simulink model "CCH_simulink"  (R2023a)
settings: Solver=VariableStepAuto  StartTime=0.0  StopTime=10.0  RelTol=1e-3
model workspace (MAT data in the model file):
  op_trim1 = opcond.OperatingReport
  op_trim1.Outputs_(1) = opcond.OutputReport
  op_trim1.Outputs_(1).yspec_ = 0
  op_trim1.Outputs_(1).Block_ = 'untitled1/Output'
  op_trim1.Outputs_(1).PortWidth_ = 1
  op_trim1.Outputs_(1).PortNumber_ = NaN
  op_trim1.Outputs_(1).Known_ = 0
  op_trim1.Outputs_(1).Min_ = -Inf
  op_trim1.Outputs_(1).Max_ = Inf
  op_trim1.Outputs_(2) = opcond.OutputReport
  op_trim1.Outputs_(2).yspec_ = 0
  op_trim1.Outputs_(2).Block_ = 'untitled1/Output1'
  op_trim1.Outputs_(2).PortWidth_ = 1
  op_trim1.Outputs_(2).PortNumber_ = NaN
  op_trim1.Outputs_(2).Known_ = 0
  op_trim1.Outputs_(2).Min_ = -Inf
  op_trim1.Outputs_(2).Max_ = Inf
  op_trim1.Outputs_(3) = opcond.OutputReport
  op_trim1.Outputs_(3).yspec_ = 0
  op_trim1.Outputs_(3).Block_ = 'untitled1/Output2'
  op_trim1.Outputs_(3).PortWidth_ = 1
  op_trim1.Outputs_(3).PortNumber_ = NaN
  op_trim1.Outputs_(3).Known_ = 0
  op_trim1.Outputs_(3).Min_ = -Inf
  op_trim1.Outputs_(3).Max_ = Inf
  op_trim1.Outputs_(4) = opcond.OutputReport
  op_trim1.Outputs_(4).yspec_ = 0
  op_trim1.Outputs_(4).Block_ = 'untitled1/Output3'
  op_trim1.Outputs_(4).PortWidth_ = 1
  op_trim1.Outputs_(4).PortNumber_ = NaN
  op_trim1.Outputs_(4).Known_ = 0
  op_trim1.Outputs_(4).Min_ = -Inf
  op_trim1.Outputs_(4).Max_ = Inf
  op_trim1.Outputs_(5) = opcond.OutputReport
  op_trim1.Outputs_(5).yspec_ = 0
  op_trim1.Outputs_(5).Block_ = 'untitled1/Output4'
  op_trim1.Outputs_(5).PortWidth_ = 1
  op_trim1.Outputs_(5).PortNumber_ = NaN
  op_trim1.Outputs_(5).Known_ = 0
  op_trim1.Outputs_(5).Min_ = -Inf
  op_trim1.Outputs_(5).Max_ = Inf
  op_trim1.TerminationString_ = 'Operating point specifications were successfully met.'
  op_trim1.OptimizationOutput_.iterations = 9
  op_trim1.OptimizationOutput_.funcCount = 115
  op_trim1.OptimizationOutput_.lssteplength = 1
  op_trim1.OptimizationOutput_.stepsize = 6.70795164914e-07
  op_trim1.OptimizationOutput_.algorithm = 'active-set'
  op_trim1.OptimizationOutput_.firstorderopt = 0
  op_trim1.OptimizationOutput_.constrviolation = 4.6916004894e-07
  op_trim1.OptimizationOutput_.message = 'Local minimum found that satisfies the constraints.
    | 
    | Optimization completed because the objective function is non-decreasing in 
    | feasible directions, to within the value of the optimality tolerance,
    | and constraints are satisfied to within the  value of the constraint tolerance.
    | 
    | <stopping criteria details>
    | 
    | Optimization completed: The first-order optimality measure, 0.000000e+00, is less
    | than options.OptimalityTolerance = 1.000000e-06, and the maximum constraint violation,
    | 4.691600e-07,is less than options.ConstraintTolerance = 1.000000e-06.'
  op_trim1.OptimizationOutput_.bestfeasible.x = [0.00151783990311; 0.004754547464; 0.000128910185441; 0.0400087459164; -0.0616136742271; -0.0892807825145; 0.340864918915; -3.49524304204e-06; 0.0478268463383]
  op_trim1.OptimizationOutput_.bestfeasible.fval = 0
  op_trim1.OptimizationOutput_.bestfeasible.constrviolation = 4.6916004894e-07
  op_trim1.OptimizationOutput_.bestfeasible.firstorderopt = 0
  op_trim1.OptimizationOutput_.progress = {'<font face="monospaced"; size=3><BR>', 'Optimizing to solve for all desired dx/dt=0, x(k+1)-x(k)=0, and y=ydes.<BR>', ' <BR>', '(Maximum Error)  Block<BR>', ' ---------------------------------------------------------<BR>', '(1.83311e+01) untitled1/CCH Dynamics/w<BR>', '(1.83310e+01) untitled1/CCH Dynamics/w<BR>', '(3.33587e+00) untitled1/CCH Dynamics/lambda_0_u<BR>', '(8.26009e-01) untitled1/CCH Dynamics/lambda_0_u<BR>', '(1.98820e-01) untitled1/CCH Dynamics/lambda_0_u<BR>', '(4.28137e-02) untitled1/CCH Dynamics/lambda_0_u<BR>', '(6.12506e-03) untitled1/CCH Dynamics/lambda_0_u<BR>', '(2.45994e-04) untitled1/CCH Dynamics/lambda_0_u<BR>', '(4.69160e-07) untitled1/CCH Dynamics/lambda_0_u<BR>', '(4.69160e-07) untitled1/CCH Dynamics/lambda_0_u<BR>', ' <BR>', 'Operating point specifications were successfully met.<BR>'}
  op_trim1.Model_ = 'untitled1'
  op_trim1.States_(1) = opcond.StateReport
  op_trim1.States_(1).dx_ = -2.49032220193e-09
  op_trim1.States_(1).Nx_ = 1
  op_trim1.States_(1).Block_ = 'untitled1/CCH Dynamics/lambda_0_p'
  op_trim1.States_(1).x_ = -0.0616136742271
  op_trim1.States_(1).SteadyState_ = 1
  op_trim1.States_(1).dxMin_ = -Inf
  op_trim1.States_(1).dxMax_ = Inf
  op_trim1.States_(1).Known_ = 0
  op_trim1.States_(1).Min_ = -Inf
  op_trim1.States_(1).Max_ = Inf
  op_trim1.States_(2) = opcond.StateReport
  op_trim1.States_(2).dx_ = -4.6916004894e-07
  op_trim1.States_(2).Nx_ = 1
  op_trim1.States_(2).Block_ = 'untitled1/CCH Dynamics/lambda_0_u'
  op_trim1.States_(2).x_ = 0.0400087459164
  op_trim1.States_(2).SteadyState_ = 1
  op_trim1.States_(2).dxMin_ = -Inf
  op_trim1.States_(2).dxMax_ = Inf
  op_trim1.States_(2).Known_ = 0
  op_trim1.States_(2).Min_ = -Inf
  op_trim1.States_(2).Max_ = Inf
  op_trim1.States_(3) = opcond.StateReport
  op_trim1.States_(3).dx_ = -3.96070598844e-12
  op_trim1.States_(3).Nx_ = 1
  op_trim1.States_(3).Block_ = 'untitled1/CCH Dynamics/q'
  op_trim1.States_(3).x_ = 0.000128910185441
  op_trim1.States_(3).SteadyState_ = 1
  op_trim1.States_(3).dxMin_ = -Inf
  op_trim1.States_(3).dxMax_ = Inf
  op_trim1.States_(3).Known_ = 0
  op_trim1.States_(3).Min_ = -Inf
  op_trim1.States_(3).Max_ = Inf
  op_trim1.States_(4) = opcond.StateReport
  op_trim1.States_(4).dx_ = 0.000128910185441
  op_trim1.States_(4).Nx_ = 1
  op_trim1.States_(4).Block_ = 'untitled1/CCH Dynamics/theta_f'
  op_trim1.States_(4).x_ = -0.0892807825145
  op_trim1.States_(4).SteadyState_ = 0
  op_trim1.States_(4).dxMin_ = -Inf
  op_trim1.States_(4).dxMax_ = Inf
  op_trim1.States_(4).Known_ = 0
  op_trim1.States_(4).Min_ = -Inf
  op_trim1.States_(4).Max_ = Inf
  op_trim1.States_(5) = opcond.StateReport
  op_trim1.States_(5).dx_ = -3.38404100297e-08
  op_trim1.States_(5).Nx_ = 1
  op_trim1.States_(5).Block_ = 'untitled1/CCH Dynamics/u'
  op_trim1.States_(5).x_ = 0.00151783990311
  op_trim1.States_(5).SteadyState_ = 1
  op_trim1.States_(5).dxMin_ = -Inf
  op_trim1.States_(5).dxMax_ = Inf
  op_trim1.States_(5).Known_ = 0
  op_trim1.States_(5).Min_ = -Inf
  op_trim1.States_(5).Max_ = Inf
  op_trim1.States_(6) = opcond.StateReport
  op_trim1.States_(6).dx_ = -9.51930090309e-10
  op_trim1.States_(6).Nx_ = 1
  op_trim1.States_(6).Block_ = 'untitled1/CCH Dynamics/w'
  op_trim1.States_(6).x_ = 0.004754547464
  op_trim1.States_(6).SteadyState_ = 1
  op_trim1.States_(6).dxMin_ = -Inf
  op_trim1.States_(6).dxMax_ = Inf
  op_trim1.States_(6).Known_ = 0
  op_trim1.States_(6).Min_ = -Inf
  op_trim1.States_(6).Max_ = Inf
  op_trim1.Inputs_(1) = opcond.InputReport
  op_trim1.Inputs_(1).Block_ = 'untitled1/Coll'
  op_trim1.Inputs_(1).PortWidth_ = 1
  op_trim1.Inputs_(1).PortDimensions_ = [1 1]
  op_trim1.Inputs_(1).u_ = 0.340864918915
  op_trim1.Inputs_(1).Known_ = 0
  op_trim1.Inputs_(1).Min_ = -Inf
  op_trim1.Inputs_(1).Max_ = Inf
  op_trim1.Inputs_(2) = opcond.InputReport
  op_trim1.Inputs_(2).Block_ = 'untitled1/LonCyc'
  op_trim1.Inputs_(2).PortWidth_ = 1
  op_trim1.Inputs_(2).PortDimensions_ = [1 1]
  op_trim1.Inputs_(2).u_ = -3.49524304204e-06
  op_trim1.Inputs_(2).Known_ = 0
  op_trim1.Inputs_(2).Min_ = -Inf
  op_trim1.Inputs_(2).Max_ = Inf
  op_trim1.Inputs_(3) = opcond.InputReport
  op_trim1.Inputs_(3).Block_ = 'untitled1/PropColl'
  op_trim1.Inputs_(3).PortWidth_ = 1
  op_trim1.Inputs_(3).PortDimensions_ = [1 1]
  op_trim1.Inputs_(3).u_ = 0.0478268463383
  op_trim1.Inputs_(3).Known_ = 0
  op_trim1.Inputs_(3).Min_ = -Inf
  op_trim1.Inputs_(3).Max_ = Inf
settings Model: Creator=prenc  LastModifiedBy=prenc
settings DataIOCC: ExternalInput=getinputstruct(op_trim1)  InitialState=getstatestruct(op_trim1)  LoadExternalInput=on  LoadInitialState=on
settings DebuggingCC: UnderSpecifiedDimensionMsg=warning

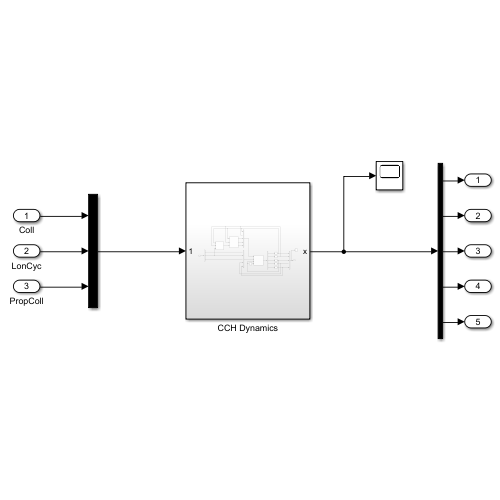
[thumbnail: Simulink's stored preview of the top-level diagram]
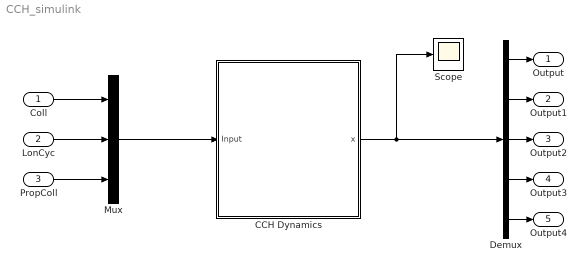
== system CCH_simulink ==
  Coll : Inport
  LonCyc : Inport  Port=2
  PropColl : Inport  Port=3
  CCH Dynamics : Subsystem
  Demux : Demux  Outputs=5
  Mux : Mux  Inputs=3
  Scope : Scope
  Output : Outport
  Output1 : Outport  Port=2
  Output2 : Outport  Port=3
  Output3 : Outport  Port=4
  Output4 : Outport  Port=5
  wires:
  LonCyc/1 -> Mux/2
  PropColl/1 -> Mux/3
  CCH Dynamics/1(x) -> Scope/1, Demux/1
  Coll/1 -> Mux/1
  Mux/1 -> CCH Dynamics/1(Input)
  Demux/1 -> Output/1
  Demux/2 -> Output1/1
  Demux/3 -> Output2/1
  Demux/4 -> Output3/1
  Demux/5 -> Output4/1

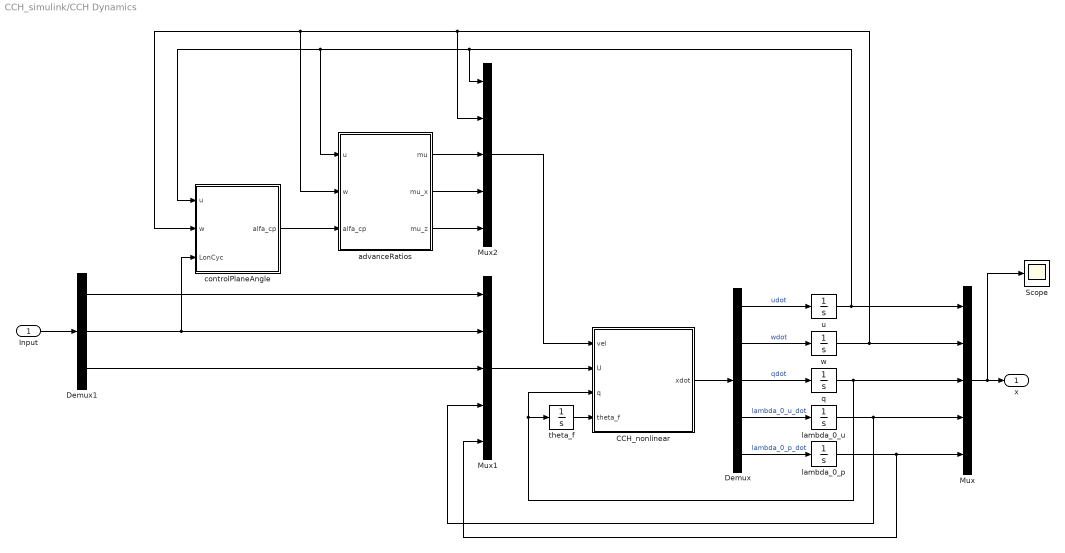
== system CCH_simulink/CCH Dynamics ==
  Input : Inport
  CCH_nonlinear : MATLAB Function  TreatAsAtomicUnit=on
  Demux : Demux  Outputs=5
  Demux1 : Demux  Outputs=3
  Mux : Mux  Inputs=5
  Mux1 : Mux  Inputs=5
  Mux2 : Mux  Inputs=5
  Scope : Scope
  advanceRatios : MATLAB Function  TreatAsAtomicUnit=on
  controlPlaneAngle : MATLAB Function  TreatAsAtomicUnit=on
  lambda_0_p : Integrator
  lambda_0_u : Integrator
  q : Integrator
  theta_f : Integrator
  u : Integrator
  w : Integrator
  x : Outport
  wires:
  advanceRatios/3(mu_z) -> Mux2/5
  Demux1/3 -> Mux1/3
  Mux1/1 -> CCH_nonlinear/2(U)
  Demux1/1 -> Mux1/1
  advanceRatios/1(mu) -> Mux2/3
  Mux2/1 -> CCH_nonlinear/1(vel)
  Demux/2 -> w/1  "wdot"
  theta_f/1 -> CCH_nonlinear/4(theta_f)
  u/1 -> Mux/1, advanceRatios/1(u), controlPlaneAngle/1(u), Mux2/1
  lambda_0_u/1 -> Mux/4, Mux1/4
  w/1 -> Mux/2, Mux2/2, advanceRatios/2(w), controlPlaneAngle/2(w)
  advanceRatios/2(mu_x) -> Mux2/4
  Demux/3 -> q/1  "qdot"
  controlPlaneAngle/1(alfa_cp) -> advanceRatios/3(alfa_cp)
  Demux1/2 -> Mux1/2, controlPlaneAngle/3(LonCyc)
  Demux/5 -> lambda_0_p/1  "lambda_0_p_dot"
  Demux/1 -> u/1  "udot"
  lambda_0_p/1 -> Mux/5, Mux1/5
  q/1 -> Mux/3, theta_f/1, CCH_nonlinear/3(q)
  Demux/4 -> lambda_0_u/1  "lambda_0_u_dot"
  Mux/1 -> Scope/1, x/1
  Input/1 -> Demux1/1
  CCH_nonlinear/1(xdot) -> Demux/1

== matlab function CCH_simulink/CCH Dynamics/advanceRatios ==
  data: u input; mu output; mu_x output; mu_z output; w input; alfa_cp input
function [mu, mu_x, mu_z] = advanceRatios(u, w, alfa_cp)

    Omega = 35;
    R = 5.49; 

    V = sqrt(u^2+w^2);
    mu = V/(Omega*R);
    mu_x = V/(Omega*R) * cos(alfa_cp);
    mu_z = V/(Omega*R) * sin(alfa_cp);

== matlab function CCH_simulink/CCH Dynamics/CCH_nonlinear ==
  data: vel input; xdot output; U input; q input; theta_f input
function xdot = CCH_nonlinear(vel, U, q, theta_f)

    %% Load helicopter parameters
    % Atmospheric Data
    g = 9.80665;
    rho = 1.225;
    
    % General Planform Data
    mass = 5500;                % Su et al. 2023
    Iyy = 16000;                % educated guess 
    CDS = 1.9;                  % Cd * S - guess from graph in report heli course assignment
    R = 5.49;                    % Su et al. 2023
    N_u = 3;
    lock = 6.57;                % Su et al. 2023
    h_l = 0.89;                 % Shaft spacing upper rotor - Su et al. 2023   
    h_u = h_l + 0.77;           % Shaft spacing lower rotor - Su et al. 2023
    hinge_offset_ratio = 0.05;
    nu_b2 = 1 + 3/2*hinge_offset_ratio/(1-hinge_offset_ratio);
    m_bl = 50;
    
    % Rotor RPM Scheduling
    
    % Main rotor Airfoil Data
    c = 0.257;                  % blade chord [m]
    c_l_a = rad2deg(0.1);       % NACA 0012
    twist_r = deg2rad(-10);
    gamma_s = deg2rad(-0);      % rotor shaft tilt
    
    % Propeller Data
    c_l_a_p = 5.7;
    omega_p = 207;  % 2300 rpm
    R_p = 1.4;
    % sigma_p = N_p*c*R_p/(pi*R_p^2);
    sigma_p = 0.142;
    Kp = 0.4;       % Downwash factor from main rotors
    l_p = 7.66;     % x location 
    h_p = 0;        % z location
    d_p = 0;        % y location
    twist_p = deg2rad(-30);
    
    % Horizontal Tail
    S_h = 5.57;
    C_l_h = 5.7;

    sigma = N_u*c*R/(pi*R^2);       % for some reason it doesnt want to read sigma from the parameters file, perhaps because of the variable name 'sigma' which is a greek letter

    %% Actual Script

    xdot = zeros(1,5);

    % Define variables for readability
    u = vel(1); w = vel(2); mu = vel(3); mu_x=vel(4); mu_z=vel(5);
    V = sqrt(u^2+w^2);
    v = 0;
    r = 0;

    alfa_fus = atan2(w,u);

    % Rotor RPM Scheduling
    if V < 70
        Omega = 40;
    else
        Omega = 40 - 5/30*(V-70);
    end

    % alfa_sp = atan2(w,u);
    % alfa_cp = alfa_sp + U(2);
    alfa_cp = U(2);

    % theta_f = deg2rad(0); 
    delta_e = 0; 

    theta_0 = U(1); theta_c = U(2); theta_p = U(3);
    lambda_0_u = U(4); lambda_0_p = U(5);

    lambda_u = (mu_z - lambda_0_u)/2;
    lambda_l = (mu_z - 2*lambda_0_u)/2;
    a0_u = lock/(8*nu_b2) * (theta_0/2*(1+mu_x^2) + 4/3*lambda_u + twist_r*(4/5+2/3*mu_x) - 4/3*mu_x*theta_c );
    a0_l = lock/(8*nu_b2) * (theta_0/2*(1+mu_x^2) + 4/3*lambda_l + twist_r*(4/5+2/3*mu_x) - 4/3*mu_x*theta_c );
    a1_u = (8/3*mu_x*theta_0/2 + 2*mu_x*lambda_u - 16/lock*q/Omega + 2*twist_r*mu_x - (1+3/2*mu_x^2)*theta_c) / (1-1/2*mu_x^2); 
    a1_l = (8/3*mu_x*theta_0/2 + 2*mu_x*lambda_l - 16/lock*q/Omega + 2*twist_r*mu_x - (1+3/2*mu_x^2)*theta_c) / (1-1/2*mu_x^2); 
    
    % H-forces
    CHdp_u = sigma*0.015*mu_x/4 + sigma*c_l_a/4*((a1_u*mu_x^2/2 + mu_x*lambda_u)*theta_0/2 ...
        + q/Omega*(-a0_u/3) + (a0_u^2+a1_u^2)*mu_x/2);
    CHdp_l = sigma*0.015*mu_x/4 + sigma*c_l_a/4*((a1_l*mu_x^2/2 + mu_x*lambda_l)*theta_0/2 ...
        + q/Omega*(-a0_l/3) + (a0_l^2+a1_l^2)*mu_x/2);

    Hdp_u = CHdp_u * rho * (Omega*R)^2 * pi*R^2;
    Hdp_l = CHdp_l * rho * (Omega*R)^2 * pi*R^2;

    % Rotor Angles
    a1r_u = theta_c - a1_u;
    a1r_l = theta_c - a1_l;

    % Thrust coefficients
    C_T_Glau_ui = 2*lambda_0_u * sqrt( (mu*cos(a1r_u))^2 + (mu*sin(a1r_u)+lambda_0_u)^2 );
    % C_T_BEM_ui = 1/4*c_l_a*sigma*(2/3*theta_0 *(1+3/2*mu_x^2)-(lambda_c+lambda_0_u));
    C_T_BEM_ui = sigma*c_l_a/2*( (1/3+mu_x^2/2)*theta_0/2 + (1+mu_x^2)/8*twist_r + lambda_u/2 );
    C_T_BEM_li = sigma*c_l_a/2*( (1/3+mu_x^2/2)*theta_0/2 + (1+mu_x^2)/8*twist_r + lambda_l/2 );

    % Thrust using BEM 
    T_u = C_T_BEM_ui * rho * (Omega*R)^2 * pi*R^2;
    % T_l = C_T_BEM_li * rho * (Omega*R)^2 * pi*R^2;
    T_l = 2*T_u;

    % Pusher Propeller Model
    alfa_sp_p = atan2(w,u);

    mu_xp = sqrt(v^2 + (w + Kp*Omega*R*(U(4)+2*U(4)) + q*l_p)^2)/(omega_p*R_p);
    lambda_p = -(u-q*h_p-r*d_p)/(omega_p*R_p) - lambda_0_p;

    C_T_Glau_p = 2*lambda_0_p*sqrt( (mu*sin(alfa_sp_p))^2 + ...
        (mu*cos(alfa_sp_p)+lambda_0_p)^2 );       % this is like climbing flight for a rotor
    C_T_BEM_p = sigma_p*c_l_a_p/2*( (1/3+mu_xp^2/2)*theta_p + (1+mu_xp^2)/8*twist_p + lambda_p/2 );
    Tp = C_T_BEM_p * rho * (omega_p*R_p)^2 * pi*R_p^2;

    % All-moving horizontal tail (elevator)
    L_h = 1/2*rho*V^2*S_h*C_l_h*(delta_e+theta_f);  % wrong, not with theta_f but with alfa_fus
    L_h = 0;  

    %% Forces and Moments
    % X Forces
    X_MR_u_H = -Hdp_u*cos(a1r_u+gamma_s);
    X_MR_u_T = T_u*sin(a1r_u+gamma_s);
    X_MR_u = X_MR_u_H + X_MR_u_T;

    X_MR_l_H = -Hdp_l*cos(a1r_l+gamma_s);
    X_MR_l_T = T_l*sin(a1r_l+gamma_s);
    X_MR_l = X_MR_l_H + X_MR_l_T;

    X_MR = X_MR_u + X_MR_l;
    X_fus = -0.5*rho*V^2*CDS*cos(alfa_fus);
    X_prop = Tp;
    X = X_MR + X_fus + X_prop;

    % Y-forces
    Y = 0;

    % Z forces
    Z_MR_u_T = -T_u*cos(a1r_u+gamma_s);
    Z_MR_l_T = -T_l*cos(a1r_l+gamma_s);
    Z_MR_u = Z_MR_u_T + Z_MR_l_T;

    Z_MR_u_H = -Hdp_u*sin(a1r_u+gamma_s);
    Z_MR_l_H = -Hdp_l*sin(a1r_l+gamma_s);
    Z_MR_l = Z_MR_u_H + Z_MR_l_H;

    Z_MR = Z_MR_u + Z_MR_l;
    Z_fus = 0.5*rho*V^2*CDS*sin(alfa_fus);
    Z_prop = 0;
    Z = Z_MR + Z_fus + Z_prop;

    % L Moment
    L = 0;

    % M Moment
    M_MR = - h_u*X_MR_u - h_l*X_MR_l;
    M_e = (Omega*R)^2*hinge_offset_ratio*m_bl*sin(a1r_u+gamma_s);    % moment due to hinge offset
    M = M_MR + M_e;

    % N Moment
    N = 0;

    %% Equations of Motion
    udot = -q*w + X/mass -g*sin(theta_f);
    wdot = q*u + Z/mass + g*cos(theta_f);
    qdot = M/Iyy;
    
    lambda_0_u_dot = (C_T_BEM_ui-C_T_Glau_ui)/0.1;
    lambda_p_dot = (C_T_BEM_p-C_T_Glau_p)/0.1;

    xdot = [udot, wdot, qdot, lambda_0_u_dot, lambda_p_dot];

end

== matlab function CCH_simulink/CCH Dynamics/controlPlaneAngle ==
  data: u input; alfa_cp output; w input; LonCyc input
function alfa_cp = controlPlaneAngle(u, w, LonCyc)

    alfa_sp = atan2(w,u);
    alfa_cp = alfa_sp + LonCyc;
